simulink model "Simulacion_CloseLoop"  (R2023b)
settings: Solver=ode4  StartTime=0.0  StopTime=10.0  FixedStep=0.001  RelTol=1e-3
undefined symbols (not defined in the file): J_p, J_r, J_y, K, K_f, K_t, V_sat
settings Model: Creator=Rafael  LastModifiedBy=Rafael

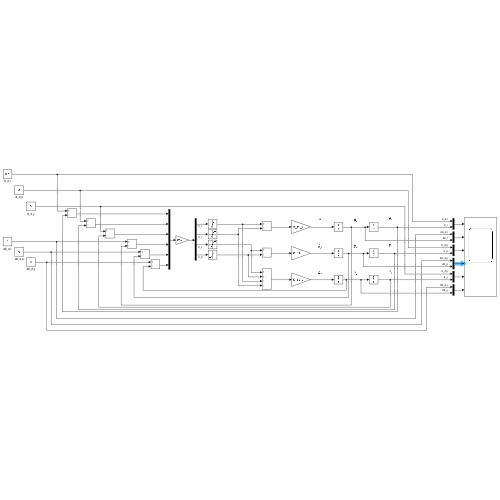
[thumbnail: Simulink's stored preview of the top-level diagram]
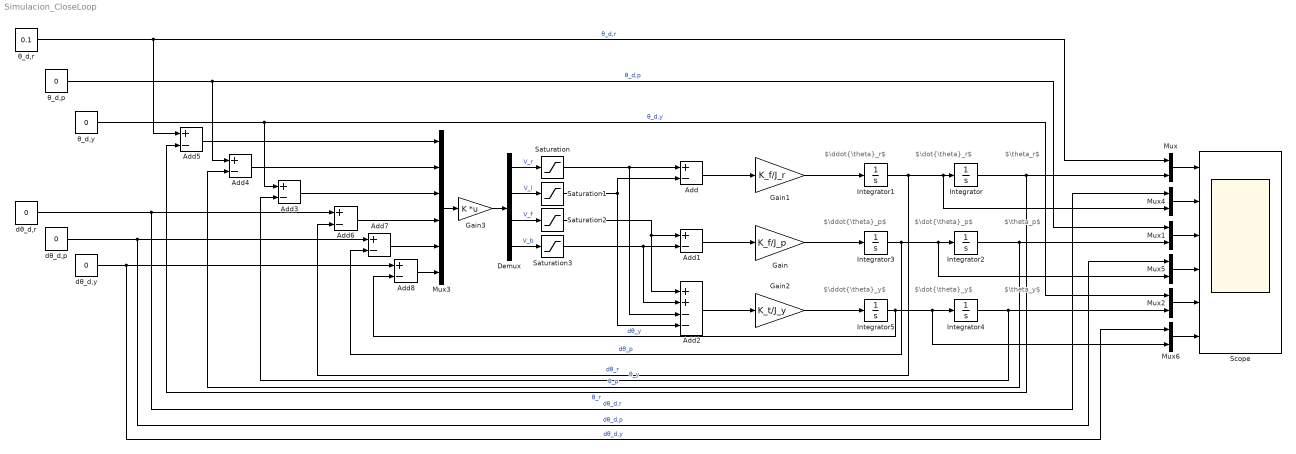
== system Simulacion_CloseLoop ==
  note: $\ddot{\theta}_r$
  note: $\dot{\theta}_r$
  note: $\dot{\theta}_p$
  note: $\ddot{\theta}_p$
  note: $\theta_p$
  note: $\theta_r$
  note: $\theta_y$
  note: $\dot{\theta}_y$
  note: $\ddot{\theta}_y$
  Add{,1,3..8} (8 alike) : Sum  Inputs=+-
  Add2 : Sum  Inputs=++--
  Demux : Demux
  Gain : Gain  Gain=K_f/J_p
  Gain1 : Gain  Gain=K_f/J_r
  Gain2 : Gain  Gain=K_t/J_y
  Gain3 : Gain  Gain=K  Multiplication=Matrix(K*u)
  Integrator{,1..5} (6 alike) : Integrator
  Mux{,1..2,4..6} (6 alike) : Mux  Inputs=2
  Mux3 : Mux  Inputs=6
  Saturation{,1..3} (4 alike) : Saturate  UpperLimit=V_sat  LowerLimit=0
  Scope : Scope  NumInputPorts=6
  dθ_d,p : Constant  Value=0
  dθ_d,r : Constant  Value=0
  dθ_d,y : Constant  Value=0
  θ_d,p : Constant  Value=0
  "θ_d,r " : Constant  Value=0.1
  θ_d,y : Constant  Value=0
  wires:
  Integrator/1 -> Add5/2, Mux/2  "θ_r"
  Integrator1/1 -> Add6/2, Mux4/2, Integrator/1  "dθ_r"
  Integrator2/1 -> Add4/2, Mux1/2  "θ_p"
  Integrator3/1 -> Add7/2, Mux5/2, Integrator2/1  "dθ_p"
  Gain/1 -> Integrator3/1
  Gain1/1 -> Integrator1/1
  Integrator4/1 -> Add3/2, Mux2/2  "θ_y"
  Gain2/1 -> Integrator5/1
  Integrator5/1 -> Add8/2, Mux6/2, Integrator4/1  "dθ_y"
  Add/1 -> Gain1/1
  Add1/1 -> Gain/1
  Add2/1 -> Gain2/1
  Demux/2 -> Saturation1/1  "V_l"
  Demux/3 -> Saturation2/1  "V_f"
  Demux/4 -> Saturation3/1  "V_b"
  Demux/1 -> Saturation/1  "V_r"
  "θ_d,r "/1 -> Mux/1, Add5/1  "θ_d,r"
  Mux/1 -> Scope/1
  Mux1/1 -> Scope/3
  Mux2/1 -> Scope/5
  θ_d,p/1 -> Add4/1, Mux1/1  "θ_d,p"
  θ_d,y/1 -> Add3/1, Mux2/1  "θ_d,y"
  Mux3/1 -> Gain3/1
  Gain3/1 -> Demux/1
  Add6/1 -> Mux3/4
  Add7/1 -> Mux3/5
  Add8/1 -> Mux3/6
  Add3/1 -> Mux3/3
  Add4/1 -> Mux3/2
  Add5/1 -> Mux3/1
  Saturation/1 -> Add2/3, Add/1
  Saturation1/1 -> Add/2, Add2/4
  Saturation2/1 -> Add1/1, Add2/1
  Saturation3/1 -> Add1/2, Add2/2
  dθ_d,p/1 -> Mux5/1, Add7/1  "dθ_d,p"
  dθ_d,y/1 -> Mux6/1, Add8/1  "dθ_d,y"
  Mux4/1 -> Scope/2
  dθ_d,r/1 -> Mux4/1, Add6/1  "dθ_d,r"
  Mux6/1 -> Scope/6
  Mux5/1 -> Scope/4
